simulink model "diff_drive"  (R2021b)
settings: Solver=VariableStepAuto  StartTime=0.0  StopTime=10.0  RelTol=1e-3
settings Model: Creator=Daniel  LastModifiedBy=Daniel

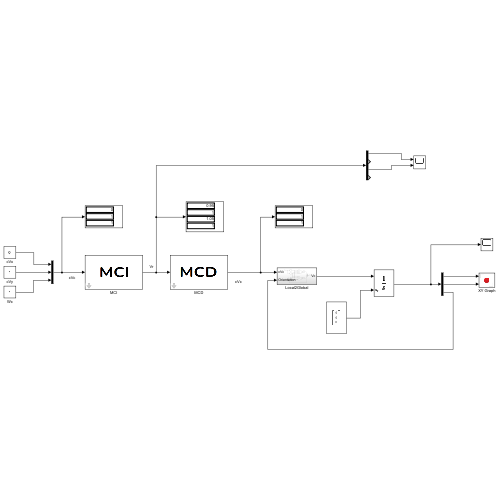
[thumbnail: Simulink's stored preview of the top-level diagram]
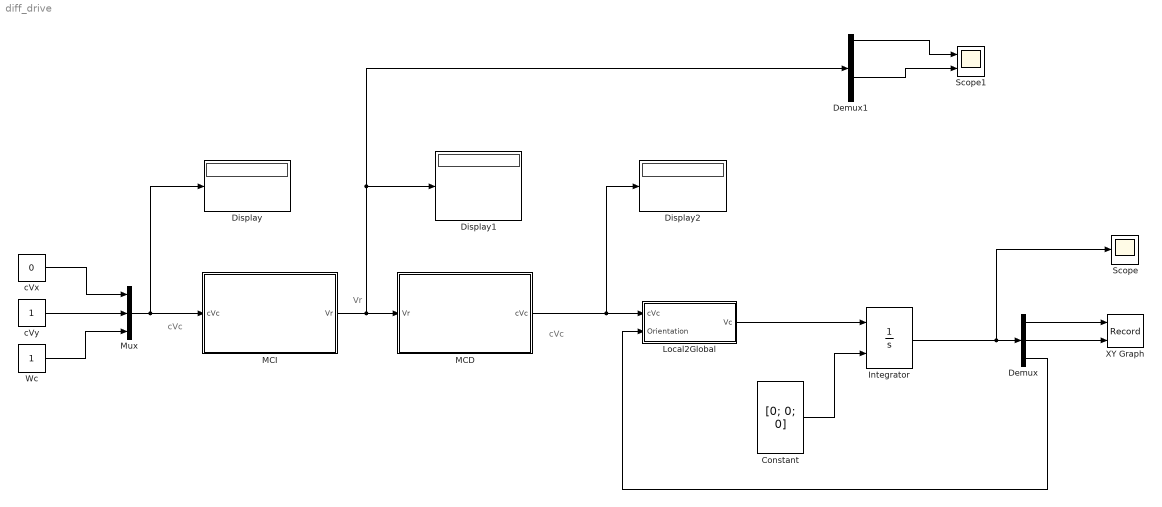
== system diff_drive ==
  note: cVc
  note: Vr
  note: cVc
  Constant : Constant  Value=[0; 0; 0]  VectorParams1D=off  SampleTime=-1
  Demux : Demux  Outputs=3
  Demux1 : Demux
  Display : Display
  Display1 : Display
  Display2 : Display
  Integrator : Integrator  InitialConditionSource=external
  Local2Global : Subsystem
  MCD : Subsystem  mask{d=0.05}
      mask prompts: d "Distancia entre ruedas"
      mask Display: image('$imagefile'); % Use "Edit Image" on toolstrip to change.
  MCI : Subsystem  mask{d=0.05}
      mask prompts: d "Distancia entre ruedas"
      mask Display: image('$imagefile'); % Use "Edit Image" on toolstrip to change.
  Mux : Mux  Inputs=3
  Scope : Scope
  Scope1 : Scope  NumInputPorts=2
  Wc : Constant
  XY Graph : Record  FileSettingsInternal="{\"entries\":[{\"content\":{\"excelSettings\":{\"content\":{},\"type\":\"Streamout.ExcelSettings\"}},\"type\":\"Streamout.FileSettingStorage\",\"uuid\":\"5f86cd49-9254-48e9-b6fa-6c42e6a2e20e\"}],\"packageUris\":[\"http://schema.mathworks.com/mf0/streamout_blocks/R2020a\"],\"version\":\"1.0\"}"  Layout=[1 1]  SignalsInternal="{\"entries\":[{\"content\":{\"signals\":[{\"content\":{\"blockPath\":[\"diff_drive/XY Graph\"],\"channel\":[],\"dimensions\":[1,1],\"domain\":\"diff_drive/XY Graph\",\"lineColor\":\"#a2142f\",\"plots\":[1],\"port\":1,\"sid\":[\"\"],\"signalID\":345,\"signalName\":\"Demux:1\"},\"type\":\"RecordBlkView.Signal\",\"uuid\":\"fdb7aa8b-154c-4a21-8f30-4fd88f7c9d8e\"},{\"content\":{\"blockPath\":[\"diff_drive/XY Graph\"],\"channel\":[],\"dimensions\":[1,1],\"domain\":\"diff_drive/XY Graph\",\"lineColor\":\"#139fff\",\"plots\":[1],\"port\":2,\"sid\":[\"\"],\"signalID\":349,\"signalName\":\"Demux:2\"},\"type\":\"RecordBlkView.Signal\",\"uuid\":\"6a517852-f632-45d9-a43d-44d1a84d97e9\"}]},\"type\":\"RecordBlkView.InputSignals\",\"uuid\":\"b6847f5e-6ef3-401d-99cc-c274a897bca5\"}],\"packageUris\":[\"http://schema.mathworks.com/mf0/streamout_blocks/R2020a\"],\"version\":\"1.0\"}"  VisualizationBindings="{\"xyplotplugin\":{\"info\":[{\"series\":[{\"bindingParametersList\":[{\"parameter\":\"X-Axis\",\"signalID\":345,\"signalName\":\"Demux:1\"},{\"parameter\":\"Y-Axis\",\"signalID\":349,\"signalName\":\"Demux:2\"}],\"seriesID\":34782}],\"subplotID\":1}]}}"  CompatibilityTag=XY
  cVx : Constant  Value=0
  cVy : Constant
  wires:
  Mux/1 -> Display/1, MCI/1(cVc)
  cVy/1 -> Mux/2
  cVx/1 -> Mux/1
  Wc/1 -> Mux/3
  Constant/1 -> Integrator/2
  Integrator/1 -> Demux/1, Scope/1
  Demux/1 -> XY Graph/1
  Demux/2 -> XY Graph/2
  MCI/1(Vr) -> Demux1/1, Display1/1, MCD/1(Vr)
  MCD/1(cVc) -> Display2/1, Local2Global/1(cVc)
  Local2Global/1(Vc) -> Integrator/1
  Demux/3 -> Local2Global/2(Orientation)
  Demux1/1 -> Scope1/1
  Demux1/3 -> Scope1/2

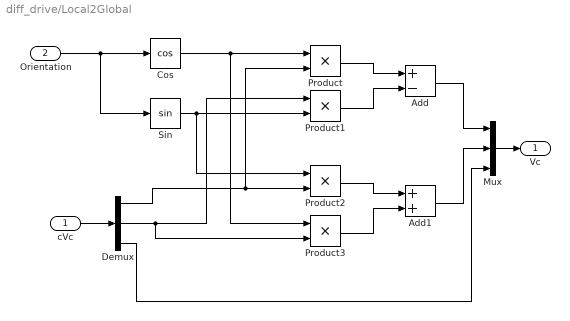
== system diff_drive/Local2Global ==
  cVc : Inport
  Orientation : Inport  Port=2
  Add : Sum  Inputs=+-
  Add1 : Sum
  Cos : Trigonometry  Operator=cos
  Demux : Demux  Outputs=3
  Mux : Mux  Inputs=3
  Product{,1..3} (4 alike) : Product
  Sin : Trigonometry
  Vc : Outport
  wires:
  Orientation/1 -> Sin/1, Cos/1
  cVc/1 -> Demux/1
  Cos/1 -> Product3/1, Product/1
  Demux/1 -> Product/2, Product2/2
  Product/1 -> Add/1
  Product2/1 -> Add1/1
  Product3/1 -> Add1/2
  Demux/2 -> Product3/2, Product1/1
  Sin/1 -> Product2/1, Product1/2
  Mux/1 -> Vc/1
  Add/1 -> Mux/1
  Add1/1 -> Mux/2
  Demux/3 -> Mux/3
  Product1/1 -> Add/2

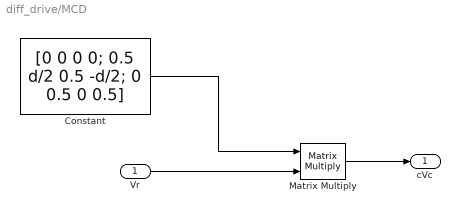
== system diff_drive/MCD ==
  Vr : Inport
  Constant : Constant  Value=[0 0 0 0; 0.5 d/2 0.5 -d/2; 0 0.5 0 0.5]  VectorParams1D=off
  Matrix Multiply : Product  Multiplication=Matrix(*)
  cVc : Outport
  wires:
  Matrix Multiply/1 -> cVc/1
  Vr/1 -> Matrix Multiply/2
  Constant/1 -> Matrix Multiply/1

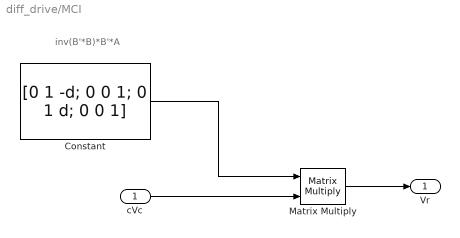
== system diff_drive/MCI ==
  note: inv(B'*B)*B'*A
  cVc : Inport
  Constant : Constant  Value=[0 1 -d; 0 0 1; 0 1 d; 0 0 1]  VectorParams1D=off
  Matrix Multiply : Product  Multiplication=Matrix(*)
  Vr : Outport
  wires:
  Matrix Multiply/1 -> Vr/1
  cVc/1 -> Matrix Multiply/2
  Constant/1 -> Matrix Multiply/1
